simulink model "mpc_rtwdemo_triggered"  (R2023a)
settings: Solver=ode3  StartTime=0.0  StopTime=10  RelTol=1e-3
values from neighbouring files (symbols this model uses):
  plant = ss(tf([3 1],[1 0.6 1]))    [mpcsubsystem1.m]
libraries: mpclib x1
settings Model: ExtModeTrigMode=oneshot  Creator=The MathWorks, Inc.  LastModifiedBy=The MathWorks, Inc.
settings SolverCC: AlgebraicLoopSolver=TrustRegion  MaxZcPerStep=1
settings DataIOCC: SaveFormat=Array  SaveOutput=off  SignalLogging=off  DSMLogging=off  SaveTime=off  ReturnWorkspaceOutputs=off  SignalLoggingName=sigsOut
settings OptimizationCC: BooleanDataType=off  ExpressionDepthLimit=2147483647  InitFltsAndDblsToZero=on  LifeSpan=inf
settings DebuggingCC: SaveWithParameterizedLinksMsg=none  UnderspecifiedInitializationDetection=Classic  MergeDetectMultiDrivingBlocksExec=none  CheckExecutionContextPreStartOutputMsg=on  SignalResolutionControl=TryResolveAllWithWarning  MultiTaskDSMMsg=warning  MultiTaskCondExecSysMsg=none  IntegerOverflowMsg=none  UnconnectedInputMsg=warning  UnconnectedOutputMsg=warning  UnconnectedLineMsg=warning  StateNameClashWarn=warning  SFUnexpectedBacktrackingDiag=warning  SFNoUnconditionalDefaultTransitionDiag=warning  SFExecutionAtInitializationDiag=none  IntegerSaturationMsg=none  ArithmeticOperatorsInVariantConditions=warning
settings HardwareCC: ProdBitPerPointer=32  ProdBitPerSizeT=32  ProdBitPerPtrDiffT=32  ProdLargestAtomicFloat=None  ProdIntDivRoundTo=Undefined  ProdEndianess=Unspecified  ProdWordSize=32  ProdHWDeviceType=32-bit Generic  TargetHWDeviceType=32-bit Generic  ProdEqTarget=off
settings ModelReferenceCC: EnableRefExpFcnMdlSchedulingChecks=on  PropagateSignalLabelsOutOfModel=off
settings SFSimCC: SimUseLocalCustomCode=off  CustomCodeUndefinedFunction=UseInterfaceOnly
settings RTWCC: RTWUseLocalCustomCode=off  DLArmComputeVersion=19.05
settings CodeAppCC: StateflowObjectComments=on
settings GRTTargetCC: TargetFcnLib=ansi_tfl_tmw.mat  TargetLangStandard=C89/C90 (ANSI)  CombineOutputUpdateFcns=off  GRTInterface=on
settings ConfigComp: CovMetricSettings=dw  CovSaveCumulativeToWorkspaceVar=on  CovSaveSingleToWorkspaceVar=on  CovExternalEMLEnable=off  CovSFcnEnable=off

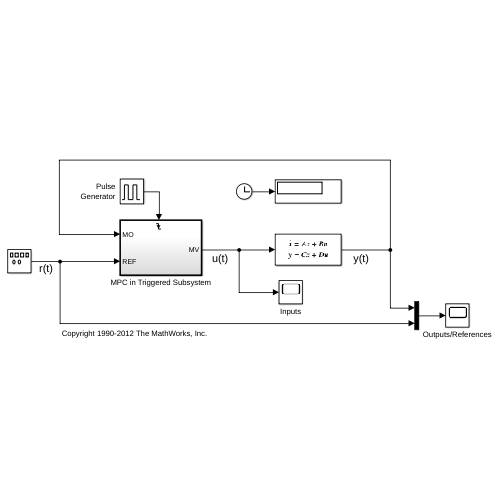
[thumbnail: Simulink's stored preview of the top-level diagram]
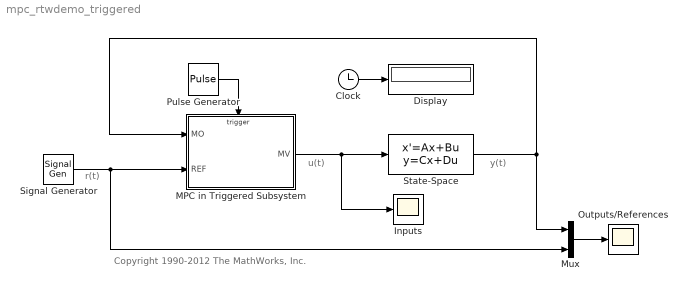
== system mpc_rtwdemo_triggered ==
  note: u(t)
  note: y(t)
  note: r(t)
  note: Copyright 1990-2012 The MathWorks, Inc.
  Clock : Clock
  Display : Display
  Inputs : Scope
  MPC in Triggered Subsystem : Subsystem
  Mux : Mux  Inputs=2
  Outputs/References : Scope
  Pulse Generator : DiscretePulseGenerator  PulseType=Time based  Period=0.1  PulseWidth=0.01  PhaseDelay=-1
  Signal Generator : SignalGenerator  Frequency=.4
  State-Space : StateSpace  A=plant.A  B=plant.B  C=plant.C  D=plant.D  InitialCondition=[0;0]
  wires:
  State-Space/1 -> Mux/1, MPC in Triggered Subsystem/1(MO)
  Mux/1 -> Outputs/References/1
  Signal Generator/1 -> Mux/2, MPC in Triggered Subsystem/2(REF)
  Clock/1 -> Display/1
  MPC in Triggered Subsystem/1(MV) -> Inputs/1, State-Space/1
  Pulse Generator/1 -> MPC in Triggered Subsystem/Trigger

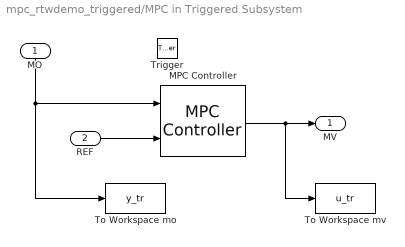
== system mpc_rtwdemo_triggered/MPC in Triggered Subsystem ==
  MO : Inport
  REF : Inport  Port=2
  Trigger : TriggerPort  TriggerType=falling  VariantControl=Variant  PortDimensions=1
  MPC Controller : mpclib/MPC Controller  mpcobj=mpcobj  x0=[]  is_multiple=0  enable_value=0  return_u0=off  updateMPCinCallerWorkspace=on  md_inport=off  mv_inport=off  uref_inport=off  return_cost=off  return_mvseq=off  return_qpstatus=off  return_xseq=off  return_state=off  return_ovseq=off  state_inport=off  umin_inport=off  umax_inport=off  ymin_inport=off  ymax_inport=off  cc_inport=off  ywt_inport=off  uwt_inport=off  duwt_inport=off  rhoeps_inport=off  pm_inport=off  MaximumP=10  HorizonChoice=FixedHorizon  n_ts=0.1  n_p=10  n_mv=1  n_md=0  n_ud=0  n_mo=1  n_uo=0  BlockDataType=double  SampleTimeInherited=on  switch_inport=off
  To Workspace mo : ToWorkspace  VariableName=y_tr  SampleTime=-1
      settings: MaxDataPoints=Inf
  To Workspace mv : ToWorkspace  VariableName=u_tr  SampleTime=-1
      settings: MaxDataPoints=Inf
  MV : Outport  VectorParamsAs1DForOutWhenUnconnected=off
  wires:
  MPC Controller/1 -> To Workspace mv/1, MV/1
  MO/1 -> To Workspace mo/1, MPC Controller/1
  REF/1 -> MPC Controller/2
